simulink model "QRLsim"  (R2013b)
settings: Solver=ode3  StartTime=0.0  StopTime=Tsim_end  FixedStep=Tsim_s  RelTol=1e-3
values from neighbouring files (symbols this model uses):
  b = 0.1    [QRLrunfile.m]    (also in hat.m = vec(2))
  b1d = [1; 0; 0]    [QRLrunfile.m]
  ctauf = 8.004e-3    (= 0.008004)    [QRLrunfile.m]
  d = 0.1    [QRLrunfile.m]
  dq0 = [0;0;0]    [QRLrunfile.m]
  dxL0 = 0    [QRLrunfile.m]
  dyL0 = 0    [QRLrunfile.m]
  dzL0 = 0    [QRLrunfile.m]
  e3 = [0;0;1]    [QRLrunfile.m]
  fsat = inf*[1 -1]    [QRLrunfile.m]
  g = 9.81    [LQRrunfile.m]    (also in QRLrunfile.m)
  I = diag([Ixx Iyy Izz])    [QRLrunfile.m]
  Ir = 0.5    [QRLrunfile.m]
  Ixx = 0.0820    (= 0.082)    [LQRrunfile.m]    (also in QRLrunfile.m = 0.00223)
  Iyy = 0.0845    [LQRrunfile.m]    (also in QRLrunfile.m = 0.00299)
  Izz = 0.1377    [LQRrunfile.m]    (also in QRLrunfile.m = 0.0048)
  K = lqr(LQRA,LQRB,LQRQ,LQRR)    [LQRrunfile.m]
  kdx = facx*3    (= 3)    [QRLrunfile.m]
  komega = 0.1    [QRLQRATT-18-Apr-2017.mat]    (also in QRLrunfile.m = 0.75; savename.mat)
  kOmega = 0.4*facR    (= 0.04)    [QRLrunfile.m]
  kpx = facx*28.5    (= 28.5)    [QRLrunfile.m]
  kq = 4    [QRLQRATT-18-Apr-2017.mat]    (also in QRLrunfile.m = 2.25; savename.mat)
  kR = 8.81    [QRLQRATT-18-Apr-2017.mat]    (also in QRLrunfile.m = 0.285; savename.mat)
  L = 0.7    [QRLrunfile.m]
  l = 0.126    [QRLrunfile.m]
  LQRA = [zeros(8) eye(8) ... (first row only)    [LQRrunfile.m]
  LQRB = [zeros(10,4) ... (first row only)    [LQRrunfile.m]
  LQRC = eye(16)    [LQRrunfile.m]
  mL = 0.1    [LQRrunfile.m]    (also in QRLrunfile.m)
  mode = 4    [QRLrunfile.m]
  mQ = 4.34    [LQRrunfile.m]    (also in QRLrunfile.m = 0.4)
  Msat = inf*[1 -1]    [QRLrunfile.m]
  phiL0 = deg2rad(0)    [QRLrunfile.m]
  pQ0 = 0    [QRLrunfile.m]
  psiL0 = 0    [QRLrunfile.m]
  q0 = [0 0 -1]    [QRLQRATT-18-Apr-2017.mat]    (also in QRLrunfile.m = Rzyx*e3*qmode; savename.mat)
  qd = [0; 0; qmode]    [QRLrunfile.m]
  qmode = -1    [QRLrunfile.m]
  qQ0 = 0    [QRLrunfile.m]
  R0 = [1  0  0; 0  0.5  -0.866025403784; 0  0.866025403784  0.5]    [QRLQRATT-18-Apr-2017.mat]    (also in QRLrunfile.m = Rzyx; savename.mat)
  Rd = eye(3)    [QRLrunfile.m]
  rQ0 = 0    [QRLrunfile.m]
  stepamp = 0.25    [QRLrunfile.m]
  stept = 1.5    [QRLrunfile.m]
  T0 = 3    [QRLrunfile.m]
  thetaL0 = deg2rad(0)    [QRLrunfile.m]
  xL0 = q0(1)*L    [QRLrunfile.m]
  yL0 = q0(2)*L    [QRLrunfile.m]
  zL0 = L+q0(3)*L    [QRLrunfile.m]
undefined symbols (not defined in the file or in its folder): lqr0, sigbuilder_block
libraries: simulink_extras x8, CF3 x7, vrlib x5, simulink x5, dspmathops x4, aerolibtransform2 x2, CommandFilter x1
(part 1 of 2)
settings Model: Creator=Nam  LastModifiedBy=Nam
settings DataIOCC: SaveFormat=StructureWithTime
settings DebuggingCC: SolverPrmCheckMsg=none

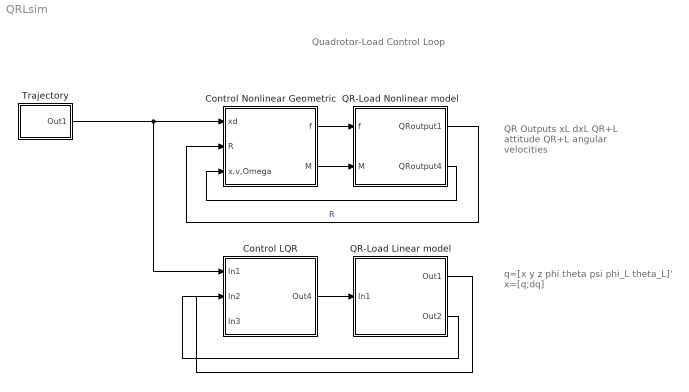
== system QRLsim ==
  note: Quadrotor-Load Control Loop
  note: QR Outputs
      | xL dxL
      | QR+L attitude
      | QR+L angular velocities
  note: q=[x y z phi theta psi phi_L theta_L]'
      | x=[q;dq]
  Control LQR : Subsystem
  Control Nonlinear Geometric : Subsystem
  QR-Load Linear model : Subsystem
  QR-Load Nonlinear model : Subsystem
  Trajectory : Subsystem
  wires:
  QR-Load Nonlinear model/1(QRoutput1) -> Control Nonlinear Geometric/2(R)  "R"
  QR-Load Nonlinear model/2(QRoutput4) -> Control Nonlinear Geometric/3(x,v,Omega)
  Control Nonlinear Geometric/1(f) -> QR-Load Nonlinear model/1(f)
  Control Nonlinear Geometric/2(M) -> QR-Load Nonlinear model/2(M)
  QR-Load Linear model/2(Out2) -> Control LQR/2(In2)
  Control LQR/1(Out4) -> QR-Load Linear model/1(In1)
  Trajectory/1(Out1) -> Control Nonlinear Geometric/1(xd), Control LQR/1(In1)
  QR-Load Linear model/1(Out1) -> ?

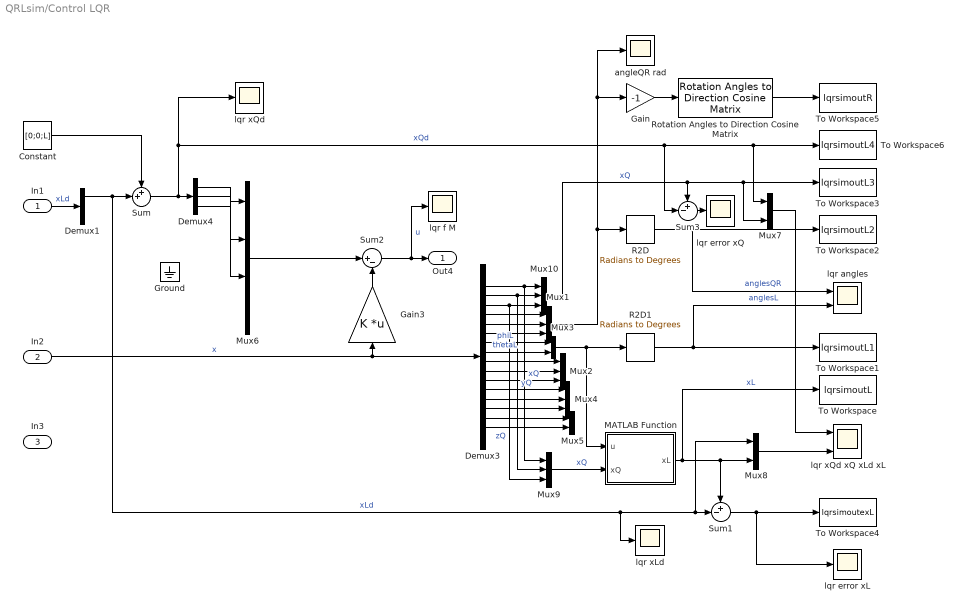
== system QRLsim/Control LQR ==
  In1 : Inport
  In2 : Inport  Port=2
  In3 : Inport  Port=3
  Constant : Constant  Value=[0;0;L]
  Demux1 : Demux  Outputs=3
  Demux3 : Demux  Outputs=16
  Demux4 : Demux  Outputs=3
  Gain : Gain  Gain=-1
  Gain3 : Gain  Gain=K  Multiplication=Matrix(K*u)
  Ground : Ground
  MATLAB Function : MATLAB Function  TreatAsAtomicUnit=on
  Mux{1..2,4,9..10} (5 alike) : Mux  Inputs=3
  Mux{3,5,7..8} (4 alike) : Mux  Inputs=2
  Mux6 : Mux
  R2D : simulink_extras/Transformations/Radians to Degrees
  R2D1 : simulink_extras/Transformations/Radians to Degrees
  Rotation Angles to Direction Cosine Matrix : aerolibtransform2/Rotation Angles to Direction Cosine Matrix  rotationOrder=XYZ
  Sum : Sum  Inputs=++|
  Sum1 : Sum  Inputs=+-|
  Sum2 : Sum  Inputs=|+-
  Sum3 : Sum  Inputs=+-|
  To Workspace : ToWorkspace  VariableName=lqrsimoutL  SampleTime=-1  SaveFormat=Structure With Time
  To Workspace1 : ToWorkspace  VariableName=lqrsimoutL1  SampleTime=-1  SaveFormat=Structure With Time
  To Workspace2 : ToWorkspace  VariableName=lqrsimoutL2  SampleTime=-1  SaveFormat=Structure With Time
  To Workspace3 : ToWorkspace  VariableName=lqrsimoutL3  SampleTime=-1  SaveFormat=Structure With Time
  To Workspace4 : ToWorkspace  VariableName=lqrsimoutexL  SampleTime=-1  SaveFormat=Structure With Time
  To Workspace5 : ToWorkspace  VariableName=lqrsimoutR  SampleTime=-1  SaveFormat=Structure With Time
  To Workspace6 : ToWorkspace  VariableName=lqrsimoutL4  SampleTime=-1  SaveFormat=Structure With Time
  angleQR rad : Scope
      settings: TimeRange=25  YMin=-0.3  YMax=1.1  SaveName=ScopeData20
  lqr angles : Scope  NumInputPorts=2
      settings: TimeRange=20  YMin=-30~-40  YMax=30~40  SaveName=ScopeData11
  lqr error xL : Scope
      settings: TimeRange=20  YMin=-1.5  YMax=2
  lqr error xQ : Scope
      settings: TimeRange=25  YMin=-0.25  YMax=0.1  SaveName=ScopeData18
  lqr f M : Scope
      settings: ShowLegends=on  SaveName=ScopeData13
  lqr xLd : Scope
      settings: TimeRange=25  YMin=-0.3  YMax=1.1  SaveName=ScopeData56
  lqr xQd : Scope
      settings: TimeRange=25  YMin=-0.25  YMax=0.1  SaveName=ScopeData58
  lqr xQd xQ xLd xL : Scope  NumInputPorts=2
      settings: ShowLegends=on  TimeRange=20  YMin=-1.5~-2  YMax=1.5~2  SaveName=ScopeData14
  Out4 : Outport
  wires:
  Constant/1 -> Sum/1
  Mux10/1 -> Mux7/2, To Workspace3/1, Sum3/1  "xQ"
  Demux1/1 -> Sum/2, lqr xLd/1, Sum1/2, Mux8/1  "xLd"
  Demux3/12 -> Mux4/1
  Demux3/14 -> Mux4/3
  Demux3/8 -> Mux3/2  "thetaL"
  Demux3/5 -> Mux1/2
  Demux3/13 -> Mux4/2
  Demux3/2 -> Mux10/2, Mux9/2  "yQ"
  Mux3/1 -> MATLAB Function/1(u), R2D1/1
  R2D/1 -> lqr angles/1, To Workspace2/1  "anglesQR"
  Sum/1 -> lqr xQd/1, Mux7/1, To Workspace6/1, Sum3/2, Demux4/1  "xQd"
  Demux3/3 -> Mux10/3, Mux9/3  "zQ"
  Mux1/1 -> angleQR rad/1, Gain/1, R2D/1
  Mux9/1 -> MATLAB Function/2(xQ)  "xQ"
  Mux6/1 -> Sum2/1
  Demux3/1 -> Mux10/1, Mux9/1  "xQ"
  MATLAB Function/1(xL) -> Sum1/1, Mux8/2, To Workspace/1  "xL"
  Demux3/15 -> Mux5/1
  Demux3/4 -> Mux1/1
  Demux3/16 -> Mux5/2
  Demux3/7 -> Mux3/1  "phiL"
  Demux3/6 -> Mux1/3
  Demux3/11 -> Mux2/3
  Demux3/10 -> Mux2/2
  Demux3/9 -> Mux2/1
  In1/1 -> Demux1/1  "xLd"
  Sum2/1 -> Out4/1, lqr f M/1  "u"
  In2/1 -> Demux3/1, Gain3/1  "x"
  Sum1/1 -> lqr error xL/1, To Workspace4/1
  R2D1/1 -> To Workspace1/1, lqr angles/2  "anglesL"
  Mux8/1 -> lqr xQd xQ xLd xL/2
  Mux7/1 -> lqr xQd xQ xLd xL/1
  Sum3/1 -> lqr error xQ/1
  Rotation Angles to Direction Cosine Matrix/1 -> To Workspace5/1
  Gain/1 -> Rotation Angles to Direction Cosine Matrix/1
  Demux4/1 -> Mux6/1
  Demux4/2 -> Mux6/2
  Demux4/3 -> Mux6/3
  Gain3/1 -> Sum2/2

== system QRLsim/Control Nonlinear Geometric ==
  note: Control
  xd : Inport
  R : Inport  Port=2
  x,v,Omega : Inport  Port=3
  QRL Load Attitude Controller : Subsystem
  QRL Load Position Controller : Subsystem
  QRL QR Attitude Controller : Subsystem
  f : Outport
  M : Outport  Port=2
  wires:
  R/1 -> QRL Load Attitude Controller/3(R), QRL QR Attitude Controller/4(R1)
  x,v,Omega/1 -> QRL Load Attitude Controller/4(QROutput), QRL QR Attitude Controller/5(Omega), QRL Load Position Controller/2(QROutput1)
  xd/1 -> QRL Load Position Controller/1(xdes)
  QRL QR Attitude Controller/1(M) -> M/1  "M"
  QRL Load Attitude Controller/2(b3d2) -> QRL QR Attitude Controller/1(R)
  QRL Load Position Controller/1(b3d1) -> QRL Load Attitude Controller/1(xdes1)
  QRL Load Position Controller/2(f) -> QRL Load Attitude Controller/2(R1)
  QRL Load Attitude Controller/1(b3d1) -> f/1  "f"
  QRL Load Attitude Controller/3(b3d3) -> QRL QR Attitude Controller/2(R2)
  QRL Load Attitude Controller/4(b3d4) -> QRL QR Attitude Controller/3(R3)

== system QRLsim/QR-Load Linear model ==
  In1 : Inport
  Gain1 : Gain  Gain=LQRA  Multiplication=Matrix(K*u)
  Gain2 : Gain  Gain=LQRB  Multiplication=Matrix(K*u)
  Gain5 : Gain  Gain=LQRC  Multiplication=Matrix(K*u)
  Integrator : Integrator  InitialCondition=lqr0
  Sum1 : Sum  Inputs=|++
  Out1 : Outport
  Out2 : Outport  Port=2
  wires:
  Gain1/1 -> Sum1/2
  Sum1/1 -> Integrator/1  "dx"
  Integrator/1 -> Gain1/1, Out2/1, Gain5/1  "x"
  Gain2/1 -> Sum1/1
  In1/1 -> Gain2/1  "u"
  Gain5/1 -> Out1/1  "y"

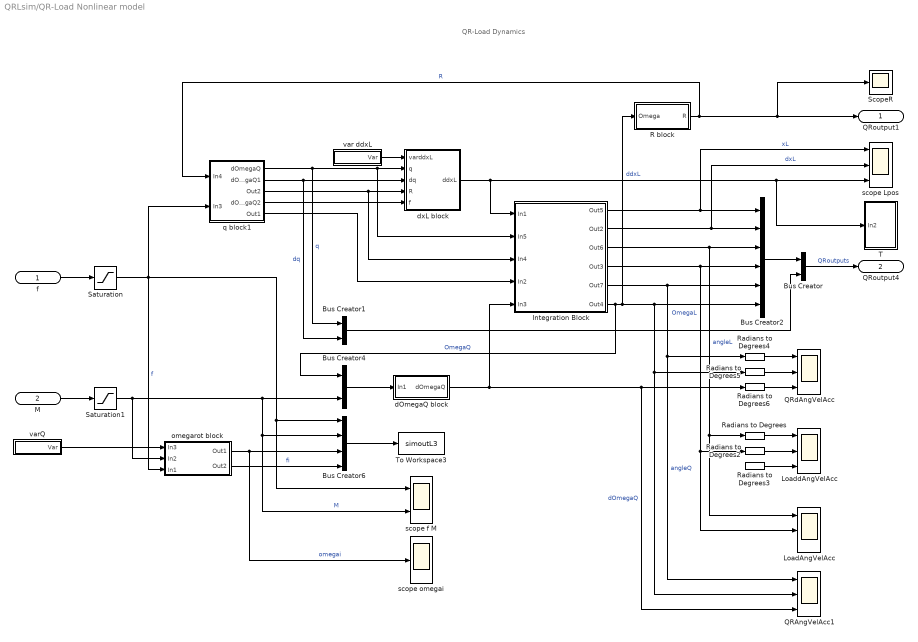
== system QRLsim/QR-Load Nonlinear model ==
  note: QR-Load Dynamics
  f : Inport
  M : Inport  Port=2  PortDimensions=3
  Bus Creator : BusCreator  Inputs=2
  Bus Creator1 : BusCreator  Inputs=2
  Bus Creator2 : BusCreator  Inputs=6
  Bus Creator4 : BusCreator  Inputs=2
  Bus Creator6 : BusCreator
  Integration Block : Subsystem
  LoadAngVelAcc : Scope  NumInputPorts=3
      settings: ShowLegends=on  YMin=-0.65~-20~-2000  YMax=0.15~12.5~1000  SaveName=ScopeData10
  LoaddAngVelAcc : Scope  NumInputPorts=3
      settings: ShowLegends=on  YMin=-5~-5~-5  YMax=5~5~5  SaveName=ScopeData4
  QRAngVelAcc1 : Scope  NumInputPorts=3
      settings: ShowLegends=on  YMin=-0.65~-20~-2000  YMax=0.15~12.5~1000  SaveName=ScopeData15
  QRdAngVelAcc : Scope  NumInputPorts=3
      settings: ShowLegends=on  TimeRange=20  YMin=-60~-600~-15000  YMax=60~800~20000  SaveName=ScopeData3
  R block : Subsystem
  Radians to Degrees{,2..6} (6 alike) : simulink_extras/Transformations/Radians to Degrees
  Saturation : Saturate  UpperLimit=fsat(1)  LowerLimit=fsat(2)
  Saturation1 : Saturate  UpperLimit=Msat(1)  LowerLimit=Msat(2)
  ScopeR : Scope
      settings: SaveName=ScopeData37
  T : Subsystem
  To Workspace3 : ToWorkspace  VariableName=simoutL3  SampleTime=-1  SaveFormat=Structure With Time
  dOmegaQ block : Subsystem
  dxL block : MATLAB Function  TreatAsAtomicUnit=on
  omegarot block : Subsystem
      mask Display: disp('(f,M) \rightarrow (\omega_i,f_i)','texmode','on')
  q block1 : Subsystem
  scope Lpos : Scope  NumInputPorts=3
      settings: ShowLegends=on  TimeRange=30  YMin=0~0~-100  YMax=7~6~250  SaveName=ScopeData12
  scope f M : Scope  NumInputPorts=2
      settings: ShowLegends=on  TimeRange=10  YMin=4.65~-2.25  YMax=5.35~1.25  SaveName=ScopeData42
  scope omegai : Scope
      settings: ShowLegends=on  YMin=42  YMax=54  SaveName=ScopeData16
  var ddxL : Subsystem
  varQ : Subsystem
  QRoutput1 : Outport
  QRoutput4 : Outport  Port=2
  wires:
  dxL block/1(ddxL) -> Integration Block/1(In1), T/1(In2), scope Lpos/3  "ddxL"
  dOmegaQ block/1(dOmegaQ) -> Integration Block/5(In3), Radians to Degrees6/1, QRAngVelAcc1/3  "dOmegaQ"
  Bus Creator4/1 -> dOmegaQ block/1(In1)
  M/1 -> Saturation1/1
  var ddxL/1(Var) -> dxL block/1(varddxL)
  q block1/2(dOmegaQ1) -> Bus Creator1/2, dxL block/3(dq)  "dq"
  q block1/3(Out2) -> dxL block/4(R), Integration Block/3(In4)
  q block1/1(dOmegaQ) -> Bus Creator1/1, Integration Block/2(In5), dxL block/2(q)  "q"
  Integration Block/5(Out7) -> Bus Creator2/5, Radians to Degrees4/1, QRAngVelAcc1/1  "angleQ"
  Integration Block/2(Out2) -> Bus Creator2/2, scope Lpos/2  "dxL"
  Integration Block/4(Out3) -> Bus Creator2/4, LoadAngVelAcc/2, Radians to Degrees2/1  "OmegaL"
  Integration Block/6(Out4) -> Bus Creator2/6, Radians to Degrees5/1, QRAngVelAcc1/2, R block/1(Omega), Bus Creator4/1  "OmegaQ"
  Integration Block/1(Out5) -> Bus Creator2/1, scope Lpos/1  "xL"
  varQ/1(Var) -> omegarot block/1(In3)
  Integration Block/3(Out6) -> Bus Creator2/3, LoadAngVelAcc/1, Radians to Degrees/1  "angleL"
  Bus Creator6/1 -> To Workspace3/1
  Radians to Degrees/1 -> LoaddAngVelAcc/1
  Radians to Degrees2/1 -> LoaddAngVelAcc/2
  Radians to Degrees3/1 -> LoaddAngVelAcc/3
  Radians to Degrees5/1 -> QRdAngVelAcc/2
  Radians to Degrees4/1 -> QRdAngVelAcc/1
  Radians to Degrees6/1 -> QRdAngVelAcc/3
  R block/1(R) -> QRoutput1/1, ScopeR/1, q block1/1(In4)  "R"
  Bus Creator1/1 -> Bus Creator/2
  Bus Creator2/1 -> Bus Creator/1
  Bus Creator/1 -> QRoutput4/1  "QRoutputs"
  q block1/5(Out1) -> Integration Block/4(In2)
  f/1 -> Saturation/1
  omegarot block/1(Out1) -> scope omegai/1, Bus Creator6/3  "omegai"
  Saturation/1 -> scope f M/1, Bus Creator6/1, q block1/2(In3), omegarot block/3(In1)  "f"
  Saturation1/1 -> omegarot block/2(In2), Bus Creator4/2, scope f M/2, Bus Creator6/2  "M"
  omegarot block/2(Out2) -> Bus Creator6/4  "fi"
  q block1/4(dOmegaQ2) -> dxL block/5(f)

== system QRLsim/Trajectory ==
  Command Filter1 : CF3/Command Filter  Integrator1_init=0  omega_n1=omega_n1_xL  omega_n2=omega_n2_xL  zeta=zeta_xL
  Ellipse : Subsystem
  Manual Switch : ManualSwitch
  Manual Switch1 : ManualSwitch
  Mux2 : Mux  Inputs=3
  Path : Subsystem
  Scope2 : Scope  NumInputPorts=3
      settings: ShowLegends=on  TimeRange=25  YMin=-0.5~-0.8~-5  YMax=2~0.6000000000000001~5
  Step : Subsystem
  Terminator : Terminator
  Out1 : Outport
  wires:
  Command Filter1/3 -> Scope2/2, Mux2/2
  Command Filter1/4 -> Scope2/3, Mux2/3
  Command Filter1/2 -> Terminator/1
  Command Filter1/1 -> Scope2/1, Mux2/1
  Mux2/1 -> Out1/1
  Manual Switch1/1 -> Command Filter1/1  "xLd"
  Step/1(Out2) -> Manual Switch/1
  Path/1(Out3) -> Manual Switch/2
  Manual Switch/1 -> Manual Switch1/1
  Ellipse/1(Out3) -> Manual Switch1/2

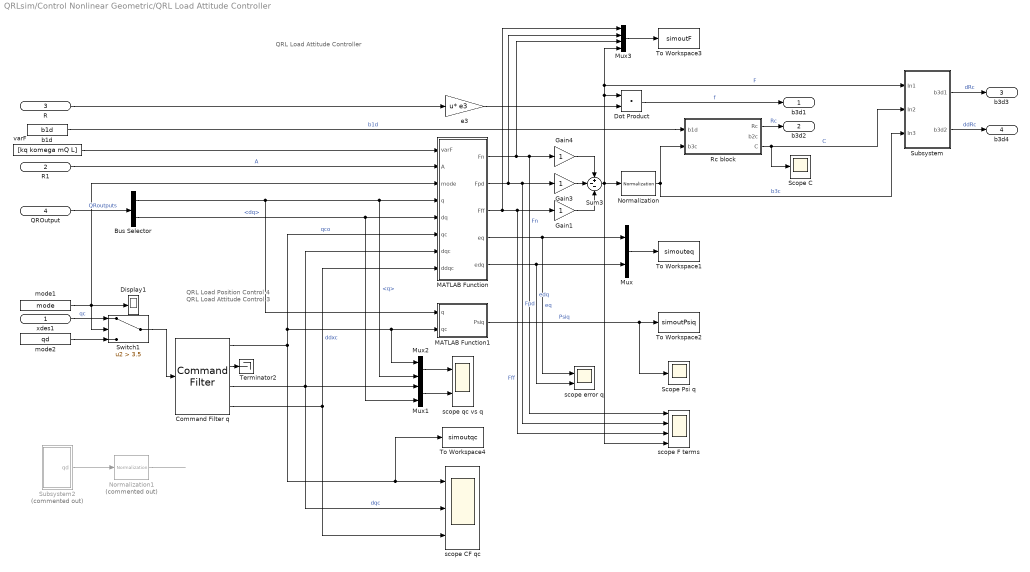
== system QRLsim/Control Nonlinear Geometric/QRL Load Attitude Controller ==
  note: QRL Load Attitude Controller
  note: QRL Load Position Control 4
      | QRL Load Attitude Control 3
  xdes1 : Inport
  R1 : Inport  Port=2
  R : Inport  Port=3
  QROutput : Inport  Port=4
  Bus Selector : BusSelector  OutputSignals=signal2.q,signal2.dq
  Command Filter q : CF3/Command Filter  Integrator1_init=q0  omega_n1=omega_n1_q  omega_n2=omega_n2_q  zeta=zeta_q
  Display1 : Display
  Dot Product : DotProduct  InputSameDT=on  OutDataTypeStr=Inherit: Inherit via internal rule
  Gain1 : Gain
  Gain3 : Gain
  Gain4 : Gain
  MATLAB Function : MATLAB Function  TreatAsAtomicUnit=on
  MATLAB Function1 : MATLAB Function  TreatAsAtomicUnit=on
  Mux : Mux  Inputs=2
  Mux1 : Mux  Inputs=2
  Mux2 : Mux  Inputs=2
  Mux3 : Mux
  Normalization : dspmathops/Normalization  NormType=2-norm  Bias=1e-10  NormOver=Each column  ColComp=on  Dimension=1  outputDataTypeStr=Inherit: Same as product output  outputLastDataTypeStr=Inherit: Same as product output  outputMin=[]  outputMax=[]  accumDataTypeStr=Inherit: Same as product output  accumLastDataTypeStr=Inherit: Same as product output  roundingMode=Floor  overflowMode=off
  Normalization1 : dspmathops/Normalization  Commented=on  NormType=2-norm  Bias=1e-10  NormOver=Each column  ColComp=on  Dimension=1  outputDataTypeStr=Inherit: Same as product output  outputLastDataTypeStr=Inherit: Same as product output  outputMin=[]  outputMax=[]  accumDataTypeStr=Inherit: Same as product output  accumLastDataTypeStr=Inherit: Same as product output  roundingMode=Floor  overflowMode=off
  Rc block : MATLAB Function  TreatAsAtomicUnit=on
  Scope C : Scope
      settings: ShowLegends=on  TimeRange=30  YMin=0  YMax=0.003  SaveName=ScopeData26
  Scope Psi q : Scope
      settings: ShowLegends=on  TimeRange=30  YMin=0  YMax=0.003  SaveName=ScopeData47
  Subsystem : Subsystem
  Subsystem2 : Subsystem  Commented=on
  Sum3 : Sum  Inputs=+--
  Switch1 : Switch  Criteria=u2 > Threshold  Threshold=3.5
  Terminator2 : Terminator
  To Workspace1 : ToWorkspace  VariableName=simouteq  SampleTime=-1  SaveFormat=Structure With Time
  To Workspace2 : ToWorkspace  VariableName=simoutPsiq  SampleTime=-1  SaveFormat=Structure With Time
  To Workspace3 : ToWorkspace  VariableName=simoutF  SampleTime=-1  SaveFormat=Structure With Time
  To Workspace4 : ToWorkspace  VariableName=simoutqc  SampleTime=-1  SaveFormat=Structure With Time
  b1d : Constant  Value=b1d  VectorParams1D=off
  e3 : Gain  Gain=e3  Multiplication=Matrix(u*K)
  mode1 : Constant  Value=mode  VectorParams1D=off
  mode2 : Constant  Value=qd  VectorParams1D=off
  scope CF qc : Scope  NumInputPorts=3
      settings: ShowLegends=on  YMin=-1~-1.5~-40  YMax=0.5~0.5~60  SaveName=ScopeData19
  scope F terms : Scope  NumInputPorts=4
      settings: TimeRange=15  YMin=-5~-5~-5~-5  YMax=5~5~5~5  SaveName=ScopeData31
  scope error q : Scope  NumInputPorts=2
      settings: TimeRange=10  YMin=-0.14~-0.5  YMax=0.06~0.5  SaveName=ScopeData33
  scope qc vs q : Scope  NumInputPorts=2
      settings: ShowLegends=on  TimeRange=10  YMin=-1~-1  YMax=0.4000000000000001~0.8  SaveName=ScopeData46
  varF : Constant  Value=[kq komega mQ L]  VectorParams1D=off
  b3d1 : Outport
  b3d2 : Outport  Port=2
  b3d3 : Outport  Port=3
  b3d4 : Outport  Port=4
  wires:
  Rc block/1(Rc) -> b3d2/1  "Rc"
  Normalization/1 -> Subsystem/3(In3), Rc block/2(b3c)  "b3c"
  b1d/1 -> Rc block/1(b1d)  "b1d"
  Sum3/1 -> Dot Product/1, Mux3/4, Subsystem/1(In1), Normalization/1, scope F terms/4  "F"
  mode1/1 -> Switch1/2, MATLAB Function/3(mode), Display1/1
  Command Filter q/1 -> MATLAB Function/6(qc), Mux2/1, MATLAB Function1/2(qc), scope CF qc/1, To Workspace4/1  "qco"
  QROutput/1 -> Bus Selector/1  "QRoutputs"
  MATLAB Function/3(Fff) -> Mux3/1, Gain1/1, scope F terms/3  "Fff"
  MATLAB Function/2(Fpd) -> Mux3/2, Gain3/1, scope F terms/2  "Fpd"
  MATLAB Function/1(Fn) -> Mux3/3, Gain4/1, scope F terms/1  "Fn"
  Bus Selector/1 -> Mux2/2, MATLAB Function/4(q), MATLAB Function1/1(q)  "<q>"
  Bus Selector/2 -> MATLAB Function/5(dq), Mux1/2  "<dq>"
  varF/1 -> MATLAB Function/1(varF)
  MATLAB Function1/1(Psiq) -> Scope Psi q/1, To Workspace2/1  "Psiq"
  Dot Product/1 -> b3d1/1  "f"
  e3/1 -> Dot Product/2
  R/1 -> e3/1
  MATLAB Function/5(edq) -> Mux/2, scope error q/2  "edq"
  MATLAB Function/4(eq) -> Mux/1, scope error q/1  "eq"
  Mux/1 -> To Workspace1/1
  R1/1 -> MATLAB Function/2(A)  "A"
  Gain1/1 -> Sum3/3
  mode2/1 -> Switch1/3
  Normalization1/1 -> ?
  Gain3/1 -> Sum3/2
  Gain4/1 -> Sum3/1
  Command Filter q/3 -> scope CF qc/2, Mux1/1, MATLAB Function/7(dqc)  "dqc"
  Command Filter q/4 -> scope CF qc/3, MATLAB Function/8(ddqc)  "ddxc"
  Mux2/1 -> scope qc vs q/1
  Mux1/1 -> scope qc vs q/2
  Subsystem2/1(qd) -> Normalization1/1
  Switch1/1 -> Command Filter q/1
  Command Filter q/2 -> Terminator2/1
  Mux3/1 -> To Workspace3/1
  xdes1/1 -> Switch1/1  "qc"
  Rc block/3(C) -> Scope C/1, Subsystem/2(In2)  "C"
  Subsystem/1(b3d1) -> b3d3/1  "dRc"
  Subsystem/2(b3d2) -> b3d4/1  "ddRc"

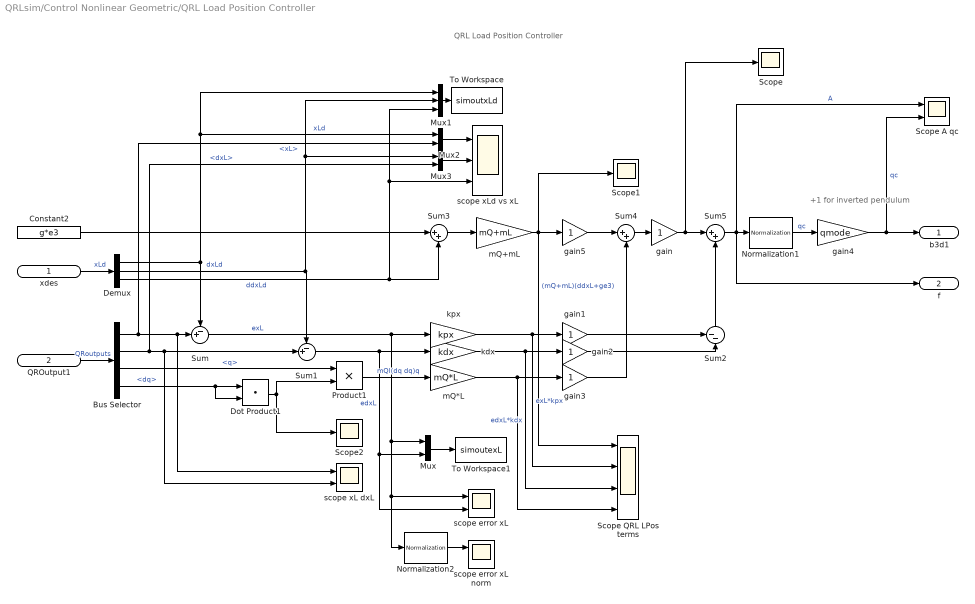
== system QRLsim/Control Nonlinear Geometric/QRL Load Position Controller ==
  note: +1 for
      | inverted pendulum
  note: QRL Load Position Controller
  xdes : Inport
  QROutput1 : Inport  Port=2
  Bus Selector : BusSelector  OutputSignals=signal1.xL,signal1.dxL,signal2.q,signal2.dq
  Constant2 : Constant  Value=g*e3
  Demux : Demux  Outputs=3
  Dot Product1 : DotProduct  InputSameDT=on  OutDataTypeStr=Inherit: Inherit via internal rule
  Mux : Mux  Inputs=2
  Mux1 : Mux  Inputs=3
  Mux2 : Mux  Inputs=2
  Mux3 : Mux  Inputs=2
  Normalization1 : dspmathops/Normalization  NormType=2-norm  Bias=1e-10  NormOver=Each column  ColComp=on  Dimension=1  outputDataTypeStr=Inherit: Same as product output  outputLastDataTypeStr=Inherit: Same as product output  outputMin=[]  outputMax=[]  accumDataTypeStr=Inherit: Same as product output  accumLastDataTypeStr=Inherit: Same as product output  roundingMode=Floor  overflowMode=off
  Normalization2 : dspmathops/Normalization  NormType=2-norm  Bias=1e-10  NormOver=Each column  ColComp=on  Dimension=1  outputDataTypeStr=Inherit: Same as product output  outputLastDataTypeStr=Inherit: Same as product output  outputMin=[]  outputMax=[]  accumDataTypeStr=Inherit: Same as product output  accumLastDataTypeStr=Inherit: Same as product output  roundingMode=Floor  overflowMode=off
  Product1 : Product
  Scope : Scope
      settings: ShowLegends=on  SaveName=ScopeData35
  Scope A qc : Scope  NumInputPorts=2
      settings: ShowLegends=on  YMin=-5~-5  YMax=5~5  SaveName=ScopeData34
  Scope QRL LPos terms : Scope  NumInputPorts=4
      settings: YMin=-5~-5~-5~-5  YMax=5~5~5~5  SaveName=ScopeData32
  Scope1 : Scope
      settings: ShowLegends=on  SaveName=ScopeData36
  Scope2 : Scope
      settings: ShowLegends=on  SaveName=ScopeData25
  Sum : Sum  Inputs=-+|
  Sum1 : Sum  Inputs=-+|
  Sum2 : Sum  Inputs=--|
  Sum3 : Sum  Inputs=|++
  Sum4 : Sum  Inputs=|++
  Sum5 : Sum  Inputs=|++
  To Workspace : ToWorkspace  VariableName=simoutxLd  SampleTime=-1  SaveFormat=Structure With Time
  To Workspace1 : ToWorkspace  VariableName=simoutexL  SampleTime=-1  SaveFormat=Structure With Time
  gain{,1..3,5} (5 alike) : Gain
  gain4 : Gain  Gain=qmode
  kdx : Gain  Gain=kdx
  kpx : Gain  Gain=kpx
  mQ*L : Gain  Gain=mQ*L
  mQ+mL : Gain  Gain=mQ+mL
  scope error xL : Scope  NumInputPorts=2
      settings: ShowLegends=on  TimeRange=10  YMin=-0.01~-0.06  YMax=0.05~0.12  SaveName=ScopeData28
  scope error xL norm : Scope  NumInputPorts=2
      settings: ShowLegends=on  TimeRange=15  YMin=-1~-200  YMax=1~275  SaveName=ScopeData57
  scope xL dxL : Scope  NumInputPorts=2
      settings: TimeRange=20  YMin=-0.5~-0.4  YMax=3.5~1.6  SaveName=ScopeData40
  scope xLd vs xL : Scope  NumInputPorts=3
      settings: ShowLegends=on  TimeRange=10  YMin=-0.025~-0.2~-0.75  YMax=0.3~0.4~0.75  SaveName=ScopeData41
  b3d1 : Outport
  f : Outport  Port=2
  wires:
  QROutput1/1 -> Bus Selector/1  "QRoutputs"
  Sum/1 -> kpx/1, Mux/1, Normalization2/1, scope error xL/1  "exL"
  Sum1/1 -> Mux/2, scope error xL/2, kdx/1  "edxL"
  Bus Selector/1 -> Mux2/2, scope xL dxL/1, Sum/2  "<xL>"
  Bus Selector/2 -> Mux3/2, scope xL dxL/2, Sum1/2  "<dxL>"
  Sum5/1 -> Scope A qc/1, f/1, Normalization1/1  "A"
  Constant2/1 -> Sum3/1
  Sum3/1 -> mQ+mL/1
  mQ+mL/1 -> gain5/1, Scope1/1, Scope QRL LPos terms/1  "(mQ+mL)(ddxL+ge3)"
  kpx/1 -> gain1/1, Scope QRL LPos terms/2  "exL*kpx"
  kdx/1 -> Scope QRL LPos terms/3, gain2/1  "edxL*kdx"
  Bus Selector/3 -> Product1/1  "<q>"
  Bus Selector/4 -> Dot Product1/2, Dot Product1/1  "<dq>"
  Dot Product1/1 -> Product1/2, Scope2/1
  Product1/1 -> mQ*L/1  "mQl(dq dq)q"
  Mux/1 -> To Workspace1/1
  Normalization1/1 -> gain4/1  "qc"
  gain3/1 -> Sum4/2
  gain4/1 -> Scope A qc/2, b3d1/1  "qc"
  gain2/1 -> Sum2/2
  gain1/1 -> Sum2/1
  Sum2/1 -> Sum5/2
  Sum4/1 -> gain/1
  gain/1 -> Scope/1, Sum5/1
  Mux1/1 -> To Workspace/1
  xdes/1 -> Demux/1  "xLd"
  Demux/1 -> Sum/1, Mux1/1, Mux2/1  "xLd"
  Demux/2 -> Mux1/2, Mux3/1, Sum1/1  "dxLd"
  Demux/3 -> Sum3/2, Mux1/3, scope xLd vs xL/3  "ddxLd"
  Mux2/1 -> scope xLd vs xL/1
  Mux3/1 -> scope xLd vs xL/2
  gain5/1 -> Sum4/1
  Normalization2/1 -> scope error xL norm/1
  mQ*L/1 -> Scope QRL LPos terms/4, gain3/1

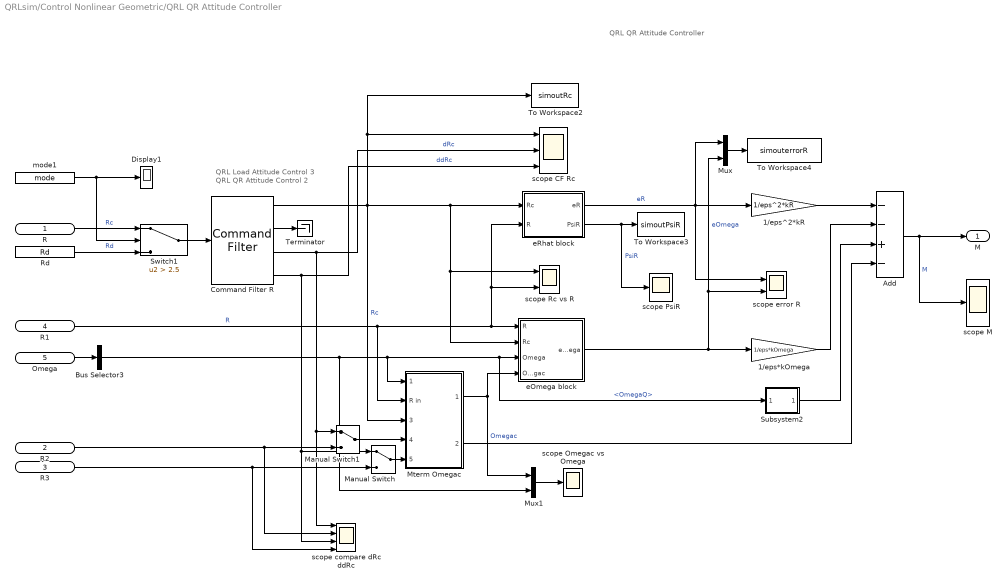
== system QRLsim/Control Nonlinear Geometric/QRL QR Attitude Controller ==
  note: QRL QR Attitude Controller
  note: QRL Load Attitude Control 3
      | QRL QR Attitude Control 2
  R : Inport
  R2 : Inport  Port=2
  R3 : Inport  Port=3
  R1 : Inport  Port=4
  Omega : Inport  Port=5
  1/eps*kOmega : Gain  Gain=1/eps*kOmega
  1/eps^2*kR : Gain  Gain=1/eps^2*kR
  Add : Sum  Inputs=--+-
  Bus Selector3 : BusSelector  OutputSignals=signal1.OmegaQ
  Command Filter R : CF3/Command Filter  Integrator1_init=R0  omega_n1=omega_n1_R  omega_n2=omega_n2_R  zeta=zeta_R
  Display1 : Display
  Manual Switch : ManualSwitch
  Manual Switch1 : ManualSwitch
  Mterm Omegac : Subsystem
  Mux : Mux  Inputs=2
  Mux1 : Mux  Inputs=2
  Rd : Constant  Value=Rd  VectorParams1D=off
  Subsystem2 : Subsystem
      mask Display: disp('\Omega \times I\Omega','texmode','on')
  Switch1 : Switch  Criteria=u2 > Threshold  Threshold=2.5
  Terminator : Terminator
  To Workspace2 : ToWorkspace  VariableName=simoutRc  SampleTime=-1  SaveFormat=Structure With Time
  To Workspace3 : ToWorkspace  VariableName=simoutPsiR  SampleTime=-1  SaveFormat=Structure With Time
  To Workspace4 : ToWorkspace  VariableName=simouterrorR  SampleTime=-1  SaveFormat=Structure With Time
  eOmega block : MATLAB Function  TreatAsAtomicUnit=on
  eRhat block : MATLAB Function  TreatAsAtomicUnit=on
  mode1 : Constant  Value=mode  VectorParams1D=off
  scope CF Rc : Scope  NumInputPorts=3
      settings: ShowLegends=on  YMin=-5~-5~-5  YMax=5~5~5  SaveName=ScopeData49
  scope M : Scope
      settings: ShowLegends=on  SaveName=ScopeData5
  scope Omegac vs Omega : Scope
      settings: ShowLegends=on  TimeRange=20  YMin=-1  YMax=1  SaveName=ScopeData51
  scope PsiR : Scope
      settings: ShowLegends=on  TimeRange=30  YMin=0  YMax=0.0025  SaveName=ScopeData44
  scope Rc vs R : Scope  NumInputPorts=2
      settings: ShowLegends=on  TimeRange=10  YMin=-0.8~-0.8  YMax=1~1  SaveName=ScopeData48
  scope compare dRc ddRc : Scope  NumInputPorts=4
      settings: ShowLegends=on  TimeRange=20  YMin=-1~-5~-5~-5  YMax=1~5~5~5  SaveName=ScopeData6
  scope error R : Scope  NumInputPorts=2
      settings: ShowLegends=on  TimeRange=10  YMin=-0.8~-4  YMax=0.6000000000000001~4  SaveName=ScopeData30
  M : Outport  PortDimensions=3
  wires:
  mode1/1 -> Switch1/2, Display1/1
  R/1 -> Switch1/1  "Rc"
  Rd/1 -> Switch1/3  "Rd"
  R1/1 -> scope Rc vs R/2, eRhat block/2(R), eOmega block/1(R), Mterm Omegac/2(R in)  "R"
  Omega/1 -> Bus Selector3/1
  Bus Selector3/1 -> Mux1/2, Mterm Omegac/1(Omega in), Subsystem2/1(Omega), eOmega block/3(Omega)  "<OmegaQ>"
  eRhat block/1(eR) -> 1/eps^2*kR/1, scope error R/1, Mux/1  "eR"
  Mterm Omegac/1(Omegades) -> Mux1/1, eOmega block/4(Omegac)  "Omegac"
  eOmega block/1(eOmega) -> 1/eps*kOmega/1, scope error R/2, Mux/2  "eOmega"
  1/eps^2*kR/1 -> Add/1
  1/eps*kOmega/1 -> Add/2
  Subsystem2/1(Out1) -> Add/3
  Mterm Omegac/2(M term) -> Add/4
  Add/1 -> scope M/1, M/1  "M"
  eRhat block/2(PsiR) -> scope PsiR/1, To Workspace3/1  "PsiR"
  Mux/1 -> To Workspace4/1
  Command Filter R/3 -> Manual Switch1/1, scope compare dRc ddRc/1, scope CF Rc/2  "dRc"
  Command Filter R/4 -> Manual Switch/1, scope compare dRc ddRc/3, scope CF Rc/3  "ddRc"
  Command Filter R/1 -> Mterm Omegac/3(Rdes in), eRhat block/1(Rc), scope Rc vs R/1, eOmega block/2(Rc), To Workspace2/1, scope CF Rc/1  "Rc"
  Mux1/1 -> scope Omegac vs Omega/1
  Switch1/1 -> Command Filter R/1
  Command Filter R/2 -> Terminator/1
  R2/1 -> Manual Switch1/2, scope compare dRc ddRc/2
  R3/1 -> Manual Switch/2, scope compare dRc ddRc/4
  Manual Switch1/1 -> Mterm Omegac/4(Rdes in1)
  Manual Switch/1 -> Mterm Omegac/5(Rdes in2)

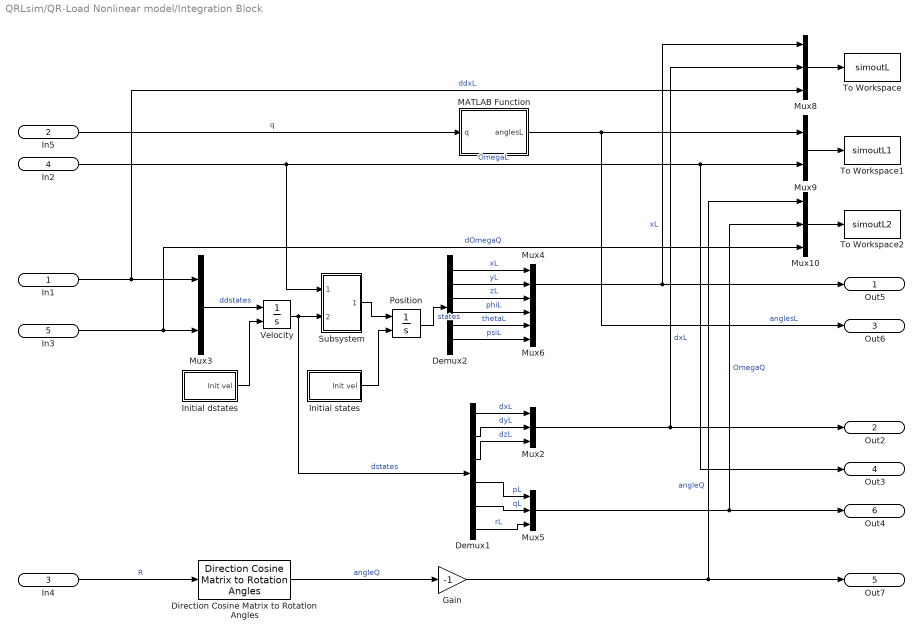
== system QRLsim/QR-Load Nonlinear model/Integration Block ==
  In1 : Inport
  In5 : Inport  Port=2
  In4 : Inport  Port=3
  In2 : Inport  Port=4
  In3 : Inport  Port=5
  Demux1 : Demux  Outputs=6
  Demux2 : Demux  Outputs=6
  Direction Cosine Matrix to Rotation Angles : aerolibtransform2/Direction Cosine Matrix to Rotation Angles  rotationOrder=XYZ  lim=Default
      settings: AttributesFormatString=Rotation Order: %<rotationOrder>
  Gain : Gain  Gain=-1
  Initial dstates : Subsystem
  Initial states : Subsystem
  MATLAB Function : MATLAB Function  TreatAsAtomicUnit=on
  Mux{2,4..6,8,10} (6 alike) : Mux  Inputs=3
  Mux3 : Mux  Inputs=2
  Mux9 : Mux  Inputs=2
  Position : Integrator  InitialConditionSource=external  ContinuousStateAttributes='position'
  Subsystem : Subsystem
  To Workspace : ToWorkspace  VariableName=simoutL  SampleTime=-1  SaveFormat=Structure With Time
  To Workspace1 : ToWorkspace  VariableName=simoutL1  SampleTime=-1  SaveFormat=Structure With Time
  To Workspace2 : ToWorkspace  VariableName=simoutL2  SampleTime=-1  SaveFormat=Structure With Time
  Velocity : Integrator  InitialConditionSource=external  ContinuousStateAttributes='velocity'
  Out5 : Outport
  Out2 : Outport  Port=2
  Out6 : Outport  Port=3
  Out3 : Outport  Port=4
  Out7 : Outport  Port=5
  Out4 : Outport  Port=6
  wires:
  In1/1 -> Mux8/3, Mux3/1  "ddxL"
  Demux1/2 -> Mux2/2  "dyL"
  Demux1/1 -> Mux2/1  "dxL"
  Demux1/3 -> Mux2/3  "dzL"
  Mux3/1 -> Velocity/1  "ddstates"
  Initial dstates/1(Init vel) -> Velocity/2
  Position/1 -> Demux2/1  "states"
  Demux2/2 -> Mux4/2  "yL"
  Demux2/1 -> Mux4/1  "xL"
  Demux2/3 -> Mux4/3  "zL"
  Initial states/1(Init vel) -> Position/2
  Demux2/4 -> Mux6/1  "phiL"
  Demux2/5 -> Mux6/2  "thetaL"
  Demux2/6 -> Mux6/3  "psiL"
  Velocity/1 -> Subsystem/2(In1), Demux1/1  "dstates"
  Mux2/1 -> Mux8/2, Out2/1  "dxL"
  Mux4/1 -> Mux8/1, Out5/1  "xL"
  In3/1 -> Mux3/2, Mux10/3  "dOmegaQ"
  Mux5/1 -> Mux10/2, Out4/1  "OmegaQ"
  Mux8/1 -> To Workspace/1
  Mux9/1 -> To Workspace1/1
  Mux10/1 -> To Workspace2/1
  In2/1 -> Subsystem/1(In2), Mux9/2, Out3/1  "OmegaL"
  Subsystem/1(Out1) -> Position/1
  Demux1/5 -> Mux5/2  "qL"
  Demux1/6 -> Mux5/3  "rL"
  Demux1/4 -> Mux5/1  "pL"
  In4/1 -> Direction Cosine Matrix to Rotation Angles/1  "R"
  Direction Cosine Matrix to Rotation Angles/1 -> Gain/1  "angleQ"
  Gain/1 -> Mux10/1, Out7/1  "angleQ"
  MATLAB Function/1(anglesL) -> Out6/1, Mux9/1  "anglesL"
  In5/1 -> MATLAB Function/1(q)  "q"

== system QRLsim/QR-Load Nonlinear model/R block ==
  note: R block
  Omega : Inport
  Integrator : Integrator  InitialCondition=R0  ContinuousStateAttributes='R'
  Saturation : Saturate  UpperLimit=1  LowerLimit=-1
  To Workspace4 : ToWorkspace  VariableName=simoutR  SampleTime=-1  SaveFormat=Structure With Time
  dR block : MATLAB Function  TreatAsAtomicUnit=on
  R : Outport
  wires:
  Integrator/1 -> Saturation/1  "R"
  dR block/1(dR) -> Integrator/1
  Omega/1 -> dR block/2(Omega)
  Saturation/1 -> dR block/1(R), To Workspace4/1, R/1  "R"

== system QRLsim/QR-Load Nonlinear model/T ==
  In2 : Inport
  Abs : Abs
  Constant : Constant  Value=g*e3
  Gain : Gain  Gain=mL
  Scope T : Scope
      settings: YMin=0  YMax=15  SaveName=ScopeData43
  Sum : Sum  Inputs=|++
  To Workspace1 : ToWorkspace  VariableName=simoutT  SampleTime=-1  SaveFormat=Structure With Time
  wires:
  Constant/1 -> Sum/2
  Abs/1 -> Scope T/1, To Workspace1/1
  Sum/1 -> Gain/1
  Gain/1 -> Abs/1
  In2/1 -> Sum/1  "ddxL"

== system QRLsim/QR-Load Nonlinear model/dOmegaQ block ==
  In1 : Inport
  Add : Sum  Inputs=-+
  Bus Selector : BusSelector  OutputSignals=OmegaQ,M
  Gain2 : Gain  Gain=inv(I)  Multiplication=Matrix(K*u)
  Subsystem1 : Subsystem
      mask Display: disp('\Omega \times I\Omega','texmode','on')
  dOmegaQ : Outport
  wires:
  In1/1 -> Bus Selector/1  "varQ"
  Bus Selector/1 -> Subsystem1/1(Omega)  "<OmegaQ>"
  Subsystem1/1(Out1) -> Add/1
  Add/1 -> Gain2/1  "J*dOmega"
  Bus Selector/2 -> Add/2  "<M>"
  Gain2/1 -> dOmegaQ/1  "dOmegaQ"

== system QRLsim/QR-Load Nonlinear model/omegarot block ==
  In3 : Inport
  In2 : Inport  Port=2
  In1 : Inport  Port=3
  Bus Selector2 : BusSelector  OutputSignals=sysvar.b,sysvar.d,sysvar.l  OutputAsBus=on
  Mux : Mux  Inputs=2
  Saturation : Saturate  UpperLimit=inf  LowerLimit=0  ZeroCross=off
  Sqrt : Sqrt  SaturateOnIntegerOverflow=on
  To Workspace3 : ToWorkspace  VariableName=simoutomegarot  SampleTime=-1  SaveFormat=Structure With Time
  fcnomega : MATLAB Function  TreatAsAtomicUnit=on
  Out1 : Outport
  Out2 : Outport  Port=2
  wires:
  In3/1 -> Bus Selector2/1
  In1/1 -> fcnomega/3(f)  "f"
  In2/1 -> fcnomega/2(M)  "M"
  Bus Selector2/1 -> fcnomega/1(var)  "var"
  Sqrt/1 -> Mux/2
  Saturation/1 -> Sqrt/1
  fcnomega/1(omegai) -> Mux/1, Saturation/1, Out1/1  "omegai"
  Mux/1 -> To Workspace3/1
  fcnomega/2(fi) -> Out2/1  "fi"

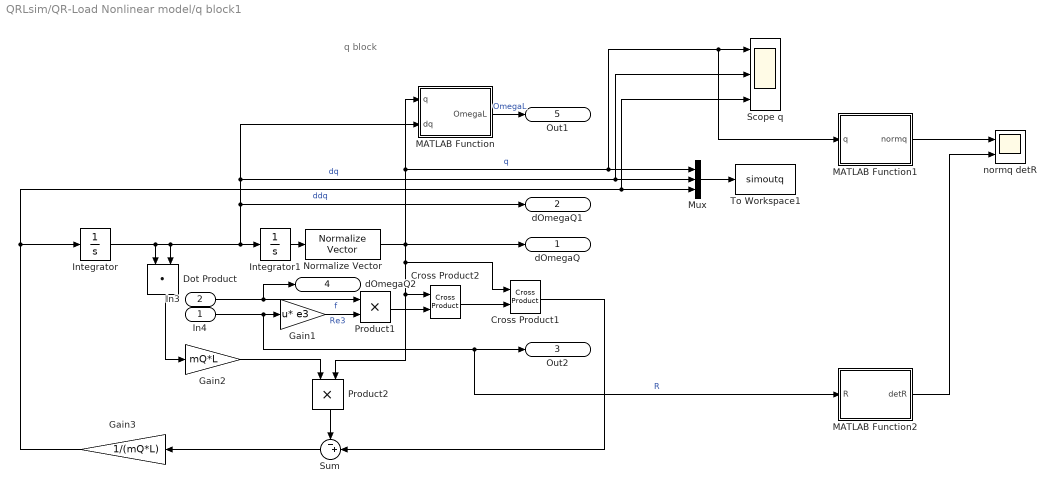
== system QRLsim/QR-Load Nonlinear model/q block1 ==
  note: q block
  In4 : Inport
  In3 : Inport  Port=2
  Cross Product1 : vrlib/Utilities/Cross Product
  Cross Product2 : vrlib/Utilities/Cross Product
  Dot Product : DotProduct  InputSameDT=on  OutDataTypeStr=Inherit: Inherit via internal rule
  Gain1 : Gain  Gain=e3  Multiplication=Matrix(u*K)
  Gain2 : Gain  Gain=mQ*L
  Gain3 : Gain  Gain=1/(mQ*L)
  Integrator : Integrator  InitialCondition=dq0  ContinuousStateAttributes='R'
  Integrator1 : Integrator  InitialCondition=q0  ContinuousStateAttributes='q'
  MATLAB Function : MATLAB Function  TreatAsAtomicUnit=on
  MATLAB Function1 : MATLAB Function  TreatAsAtomicUnit=on
  MATLAB Function2 : MATLAB Function  TreatAsAtomicUnit=on
  Mux : Mux  Inputs=3
  Normalize Vector : vrlib/Utilities/Normalize Vector  maxzero=0
  Product1 : Product
  Product2 : Product
  Scope q : Scope  NumInputPorts=3
      settings: ShowLegends=on  TimeRange=20  YMin=-1~-0.005~-0.75  YMax=0.1~0.04~1.75  SaveName=ScopeData39
  Sum : Sum  Inputs=-+|
  To Workspace1 : ToWorkspace  VariableName=simoutq  SampleTime=-1  SaveFormat=Structure With Time
  normq detR : Scope  NumInputPorts=2
      settings: YMin=-5~-5  YMax=5~5  SaveName=ScopeData29
  dOmegaQ : Outport
  dOmegaQ1 : Outport  Port=2
  Out2 : Outport  Port=3
  dOmegaQ2 : Outport  Port=4
  Out1 : Outport  Port=5
  wires:
  Dot Product/1 -> Gain2/1
  Gain3/1 -> Scope q/3, Mux/3, Integrator/1  "ddq"
  Integrator/1 -> Dot Product/1, Dot Product/2, Integrator1/1, dOmegaQ1/1, Scope q/2, Mux/2, MATLAB Function/2(dq)  "dq"
  In3/1 -> dOmegaQ2/1, Product1/1  "f"
  Gain1/1 -> Product1/2  "Re3"
  Product1/1 -> Cross Product2/2
  Cross Product2/1 -> Cross Product1/2
  Cross Product1/1 -> Sum/2
  Sum/1 -> Gain3/1
  In4/1 -> MATLAB Function2/1(R), Out2/1, Gain1/1  "R"
  Gain2/1 -> Product2/1
  Product2/1 -> Sum/1
  MATLAB Function/1(OmegaL) -> Out1/1  "OmegaL"
  Mux/1 -> To Workspace1/1
  Normalize Vector/1 -> MATLAB Function1/1(q), Scope q/1, Mux/1, MATLAB Function/1(q), dOmegaQ/1, Cross Product2/1, Product2/2, Cross Product1/1  "q"
  MATLAB Function1/1(normq) -> normq detR/1
  MATLAB Function2/1(detR) -> normq detR/2
  Integrator1/1 -> Normalize Vector/1

== system QRLsim/QR-Load Nonlinear model/var ddxL ==
  Bus Creator1 : BusCreator
  Cable length : Constant  Value=L
  Gravity Constant : Constant  Value=g
  Mass Load : Constant  Value=mL
  Mass QR : Constant  Value=mQ
  Var : Outport
  wires:
  Mass QR/1 -> Bus Creator1/1  "mQ"
  Cable length/1 -> Bus Creator1/4  "L"
  Mass Load/1 -> Bus Creator1/3  "mL"
  Bus Creator1/1 -> Var/1  "varddxL"
  Gravity Constant/1 -> Bus Creator1/2  "g"

== system QRLsim/QR-Load Nonlinear model/varQ ==
  Arm length : Constant  Value=l
  Bus Creator : BusCreator  Inputs=2
  Bus Creator1 : BusCreator  Inputs=8
  Cable length : Constant  Value=L
  Drag Factor : Constant  Value=d
  Gravity Constant : Constant  Value=g
  Mass QR : Constant  Value=mQ
  QR Inertia : Constant  Value=diag([Ixx,Iyy,Izz])
  Rotor Inertia : Constant  Value=Ir
  Thrust Factor : Constant  Value=b
  ctauf : Constant  Value=ctauf
      mask Display: disp('c_{\tau f}','texmode','on')
  Var : Outport
  wires:
  Gravity Constant/1 -> Bus Creator/2  "g"
  Bus Creator/1 -> Var/1  "varQ"
  Mass QR/1 -> Bus Creator1/1  "m"
  Arm length/1 -> Bus Creator1/6  "l"
  Rotor Inertia/1 -> Bus Creator1/5  "Ir"
  QR Inertia/1 -> Bus Creator1/2  "I"
  Bus Creator1/1 -> Bus Creator/1  "sysvar"
  Thrust Factor/1 -> Bus Creator1/3  "b"
  Drag Factor/1 -> Bus Creator1/4  "d"
  ctauf/1 -> Bus Creator1/7  "ctauf"
  Cable length/1 -> Bus Creator1/8  "lL"

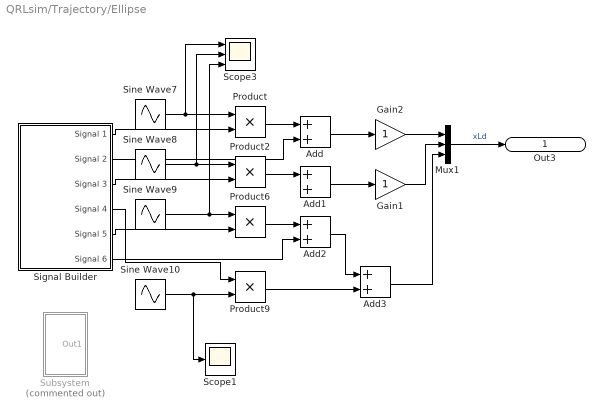
== system QRLsim/Trajectory/Ellipse ==
  Add{,1..3} (4 alike) : Sum
  Gain1 : Gain
  Gain2 : Gain
  Mux1 : Mux  Inputs=3
  Product{,2,6,9} (4 alike) : Product
  Scope1 : Scope
      settings: ShowLegends=on  YMin=-8  YMax=12  SaveName=ScopeData2
  Scope3 : Scope  NumInputPorts=3
      settings: TimeRange=25  YMin=0~0~0  YMax=2~0.5~0.5  SaveName=ScopeData23
  Signal Builder : Subsystem  Tag=STV Subsys  LoadFcn=sigbuilder_block('load');  StartFcn=sigbuilder_block('start');  StopFcn=sigbuilder_block('stop');  ClipboardFcn=sigbuilder_block('clipboard');  mask(Sigbuilder block){}
      mask help: Simulink:masks:SigbuilderBlock_MD
      mask init:
      | if ~strcmp(get_param(bdroot(gcbh),'SimulationStatus'),'stopped') tuvar = sigbuilder_block('maskInit'); end
      settings: CopyFcn=sigbuilder_block('copy');  DeleteFcn=sigbuilder_block('delete');  ModelCloseFcn=sigbuilder_block('modelClose');  PreSaveFcn=sigbuilder_block('preSave');  PauseFcn=sigbuilder_block('pause');  ContinueFcn=sigbuilder_block('continue');  NameChangeFcn=sigbuilder_block('namechange');  OpenFcn=sigbuilder_block('open',[-24 211.5 948 480 ]);  CloseFcn=sigbuilder_block('close');
      mask Display: plot(0, 0, 100, 100,[2, 2, 32, 32, 2], [68, 8, 8, 68, 68],[32, 2], [38, 38], [32, 19, 2],[53, 60, 44], [32, 17, 17, 2],[16, 16, 31, 31]);txt = getActiveGroup(gcbh);text(2, 100, txt,'verticalAlignment', 'top');
  Sine Wave10 : Sin  Amplitude=0.125  Bias=-.125  Frequency=2*pi/3  Phase=0.5*pi  SampleTime=0
  Sine Wave7 : Sin  Bias=1  Frequency=2*pi/20  Phase=pi  SampleTime=0
  Sine Wave8 : Sin  Amplitude=.4  Bias=.4  Frequency=2*pi/3  SampleTime=0
  Sine Wave9 : Sin  Amplitude=0.25  Frequency=2*pi/3  Phase=0.5*pi  SampleTime=0
  Subsystem : Subsystem  Commented=on
  Out3 : Outport
  wires:
  Add3/1 -> Mux1/3
  Gain1/1 -> Mux1/2
  Gain2/1 -> Mux1/1
  Sine Wave7/1 -> Product/1, Scope3/1
  Product/1 -> Add/1
  Signal Builder/1(Signal 1) -> Product/2
  Signal Builder/2(Signal 2) -> Add/2
  Signal Builder/3(Signal 3) -> Product2/2
  Signal Builder/5(Signal 5) -> Product6/2
  Product2/1 -> Add1/1
  Product6/1 -> Add2/1
  Add/1 -> Gain2/1
  Add1/1 -> Gain1/1
  Add2/1 -> Add3/1
  Sine Wave8/1 -> Product2/1, Scope3/2
  Sine Wave9/1 -> Scope3/3, Product6/1
  Mux1/1 -> Out3/1  "xLd"
  Signal Builder/6(Signal 6) -> Add2/2
  Signal Builder/4(Signal 4) -> Product9/1
  Sine Wave10/1 -> Scope1/1, Product9/2
  Product9/1 -> Add3/2

== system QRLsim/Trajectory/Path ==
  Manual Switch : ManualSwitch
  Sines : Subsystem
  Square : Subsystem
  Out3 : Outport
  wires:
  Square/1(Out1) -> Manual Switch/2
  Sines/1(Out1) -> Manual Switch/1
  Manual Switch/1 -> Out3/1  "xLd"

== system QRLsim/Trajectory/Step ==
  Manual Switch : ManualSwitch
  step1dir : Subsystem  mask{stept=stept, stepamp=stepamp}
      mask prompts: stept "Step time"; stepamp "Step Amplitude"
  step3dir : Subsystem
  Out2 : Outport
  wires:
  Manual Switch/1 -> Out2/1  "xLd"
  step3dir/1(Out1) -> Manual Switch/2
  step1dir/1(Out1) -> Manual Switch/1

== system QRLsim/Control Nonlinear Geometric/QRL Load Attitude Controller/Subsystem ==
  In1 : Inport
  In2 : Inport  Port=2
  In3 : Inport  Port=3
  Command Filter q1 : CF3/Command Filter  Integrator1_init=(mQ+mL)*(g*e3)  omega_n1=100  omega_n2=100  zeta=zeta_q
  Command Filter q2 : CF3/Command Filter  Integrator1_init=[0;-1;0]  omega_n1=100  omega_n2=100  zeta=zeta_q
  MATLAB Function : MATLAB Function  TreatAsAtomicUnit=on
  b3d1 : Outport
  b3d2 : Outport  Port=2
  wires:
  In1/1 -> Command Filter q1/1  "F"
  In2/1 -> Command Filter q2/1  "C"
  Command Filter q1/2 -> ?
  Command Filter q2/2 -> ?
  Command Filter q2/1 -> MATLAB Function/1(C)
  Command Filter q2/3 -> MATLAB Function/2(dC)
  Command Filter q2/4 -> MATLAB Function/3(ddC)
  Command Filter q1/1 -> MATLAB Function/5(F)
  Command Filter q1/3 -> MATLAB Function/6(dF)
  Command Filter q1/4 -> MATLAB Function/7(ddF)
  In3/1 -> MATLAB Function/4(b3c)  "b3c"
  MATLAB Function/1(dRc) -> b3d1/1  "dRc"
  MATLAB Function/2(ddRc) -> b3d2/1  "ddRc"

== system QRLsim/Control Nonlinear Geometric/QRL Load Attitude Controller/Subsystem2 ==
  Gain : Gain
  Mux2 : Mux  Inputs=3
  Product2 : Product
  Product5 : Product
  Product6 : Product
  Scope qd : Scope  NumInputPorts=2
      settings: YMin=-5~-5  YMax=5~5  SaveName=ScopeData38
  Sine Wave5 : Sin  Amplitude=.5  Frequency=2*pi/5  SampleTime=0
  Sine Wave6 : Sin  Amplitude=.5  Frequency=2*pi/5  Phase=pi/2  SampleTime=0
  Step2 : Step  Time=15  Before=1  After=0  SampleTime=0
  Step3 : Step  Time=15  Before=1  After=0  SampleTime=0
  Step4 : Step  Time=12.5  Before=-.85  After=-1  SampleTime=0
  qd : Outport
  wires:
  Sine Wave6/1 -> Product6/2
  Sine Wave5/1 -> Product5/2
  Step2/1 -> Product6/1, Product5/1
  Product5/1 -> Scope qd/2, Mux2/2
  Product6/1 -> Gain/1
  Gain/1 -> Product2/1
  Step3/1 -> Product2/2
  Product2/1 -> Scope qd/1, Mux2/1
  Mux2/1 -> qd/1  "qd"
  Step4/1 -> Mux2/3

== system QRLsim/Control Nonlinear Geometric/QRL QR Attitude Controller/Mterm Omegac ==
  Omega in : Inport
  R in : Inport  Port=2
  Rdes in : Inport  Port=3
  Rdes in1 : Inport  Port=4
  Rdes in2 : Inport  Port=5
  CFOmega : CommandFilter/Command Filter  Integrator1_init=0  omega_n=2*pi*15  zeta=.95
  Mux : Mux  Inputs=2
  Omegac block : MATLAB Function  TreatAsAtomicUnit=on
  Scope : Scope
      settings: ShowLegends=on  SaveName=ScopeData9
  Subsystem1 : Subsystem
      mask Display: disp('J_Q(\Omega^{hat}R^TR_c\Omega_c-R^TR_d\Omega\prime_c)','texmode','on')
  Terminator : Terminator
  Terminator1 : Terminator
  scope Omega Omegac : Scope  NumInputPorts=3
      settings: ShowLegends=on  YMin=-8~-5.5~-90  YMax=8~5.5~90  SaveName=ScopeData22
  Omegades : Outport
  M term : Outport  Port=2
  wires:
  Omega in/1 -> scope Omega Omegac/1, Subsystem1/2(In2)  "Omega"
  Omegac block/1(Omegac) -> CFOmega/1, scope Omega Omegac/2, Subsystem1/4(In4), Omegades/1  "Omegac"
  R in/1 -> Subsystem1/1(In1)  "R"
  Subsystem1/1(Out1) -> M term/1
  Rdes in/1 -> Subsystem1/3(In3), Omegac block/1(Rc)
  Rdes in2/1 -> Omegac block/3(ddRc)
  Rdes in1/1 -> Omegac block/2(dRc)
  CFOmega/2 -> Terminator/1
  CFOmega/1 -> Terminator1/1
  Mux/1 -> Scope/1
  Omegac block/2(dOmegac) -> scope Omega Omegac/3, Subsystem1/5(In5), Mux/2  "dOmegac"
  CFOmega/3 -> Mux/1  "CFdOmegac"

== system QRLsim/Control Nonlinear Geometric/QRL QR Attitude Controller/Subsystem2 ==
  Omega : Inport
  Cross Product : vrlib/Utilities/Cross Product
  I : Gain  Gain=I  Multiplication=Matrix(K*u)
  Out1 : Outport
  wires:
  Omega/1 -> Cross Product/1, I/1
  I/1 -> Cross Product/2
  Cross Product/1 -> Out1/1

== system QRLsim/QR-Load Nonlinear model/Integration Block/Initial dstates ==
  Bus Creator1 : BusCreator  Inputs=2
  OmegaQ0 : Constant  Value=[pQ0; qQ0; rQ0]
  dxL0 : Constant  Value=[dxL0;dyL0;dzL0]
  Init vel : Outport
  wires:
  dxL0/1 -> Bus Creator1/1  "dxL0"
  Bus Creator1/1 -> Init vel/1  "Init dstates"
  OmegaQ0/1 -> Bus Creator1/2  "OmegaQ0"

== system QRLsim/QR-Load Nonlinear model/Integration Block/Initial states ==
  Bus Creator1 : BusCreator  Inputs=2
  angleL0 : Constant  Value=[phiL0; thetaL0; psiL0]
  xL0 : Constant  Value=[xL0;yL0;zL0]
  Init vel : Outport
  wires:
  xL0/1 -> Bus Creator1/1  "xL0"
  Bus Creator1/1 -> Init vel/1  "Init states"
  angleL0/1 -> Bus Creator1/2  "angleL0"

== system QRLsim/QR-Load Nonlinear model/Integration Block/Subsystem ==
  In2 : Inport
  In1 : Inport  Port=2
  Demux3 : Demux  Outputs=6
  Mux11 : Mux
  Out1 : Outport
  wires:
  Mux11/1 -> Out1/1
  In1/1 -> Demux3/1
  Demux3/2 -> Mux11/2
  Demux3/1 -> Mux11/1
  Demux3/3 -> Mux11/3
  In2/1 -> Mux11/4

== system QRLsim/QR-Load Nonlinear model/dOmegaQ block/Subsystem1 ==
  Omega : Inport
  Cross Product : vrlib/Utilities/Cross Product
  I : Gain  Gain=I  Multiplication=Matrix(K*u)
  Out1 : Outport
  wires:
  Omega/1 -> Cross Product/1, I/1
  I/1 -> Cross Product/2
  Cross Product/1 -> Out1/1

== system QRLsim/Trajectory/Ellipse/Signal Builder ==
  Demux : Demux  Tag=STV Demux  Outputs=6
  FromWs : FromWorkspace  Tag=STV FromWs  VariableName=tuvar  SampleTime=0
      SigBuilderData=|
      | common.afterFinalStr = 'Extrapolate'
      | common.sampleTime = 0
      | dataSet.timeRange = [0 21]
      | dataSet.name = 'Group 1'
      | sbobj.Groups.Name = 'Group 1'
      | sbobj.Groups.Signals(1).Name = 'Signal 1'
      | sbobj.Groups.Signals(1).XData = [0 5 5 15 15 21]
      | sbobj.Groups.Signals(1).YData = [0 0 1 1 0 0]
      | sbobj.Groups.Signals(2).Name = 'Signal 2'
      | sbobj.Groups.Signals(2).XData = [0 15 15 21]
      | sbobj.Groups.Signals(2).YData = [0 0 2 2]
      | sbobj.Groups.Signals(3).Name = 'Signal 3'
      | sbobj.Groups.Signals(3).XData = [0 5.25 5.25 14.25 14.25 21]
      | sbobj.Groups.Signals(3).YData = [0 0 1 1 0 0]
      | sbobj.Groups.Signals(4).Name = 'Signal 4'
      | sbobj.Groups.Signals(4).XData = [0 1.5 1.5 21]
      | sbobj.Groups.Signals(4).YData = [1 1 0 0]
      | sbobj.Groups.Signals(5).Name = 'Signal 5'
      | sbobj.Groups.Signals(5).XData = [0 4.5 4.5 15 15 21]
      | sbobj.Groups.Signals(5).YData = [0 0 1 1 0 0]
      | sbobj.Groups.Signals(6).Name = 'Signal 6'
      | sbobj.Groups.Signals(6).XData = [0 1.5 1.5 4.5 4.5 15 15 21]
      | sbobj.Groups.Signals(6).YData = [0 0 -0.25 -0.25 0 0 0.25 0.25]
      | sbobj.Groups.TimeRange = [0 21]
  Signal 1 : Outport  Tag=STV Outport
  Signal 2 : Outport  Tag=STV Outport  Port=2
  Signal 3 : Outport  Tag=STV Outport  Port=3
  Signal 4 : Outport  Tag=STV Outport  Port=4
  Signal 5 : Outport  Tag=STV Outport  Port=5
  Signal 6 : Outport  Tag=STV Outport  Port=6
  wires:
  FromWs/1 -> Demux/1
  Demux/1 -> Signal 1/1
  Demux/2 -> Signal 2/1
  Demux/3 -> Signal 3/1
  Demux/4 -> Signal 4/1
  Demux/5 -> Signal 5/1
  Demux/6 -> Signal 6/1

== system QRLsim/Trajectory/Ellipse/Subsystem ==
  Constant : Constant  Value=0
  Constant1 : Constant
  Manual Switch1 : ManualSwitch
  Manual Switch2 : ManualSwitch
  Manual Switch3 : ManualSwitch
  Mux : Mux  Inputs=3
  Ramp : simulink/Sources/Ramp  slope=1/5  start=2  X0=0
  Ramp1 : simulink/Sources/Ramp  slope=0  start=0  X0=0
  Ramp2 : simulink/Sources/Ramp  slope=0  start=0  X0=0
  Sine Wave : Sin  Frequency=2*pi/T0  Phase=-pi/2  SampleTime=0
  Sine Wave3 : Sin  Frequency=2*pi/T0  SampleTime=0
  Sum2 : Sum  Inputs=|++
  Sum4 : Sum  Inputs=|++
  Out1 : Outport
  wires:
  Constant/1 -> Manual Switch1/2, Manual Switch3/2
  Sine Wave3/1 -> Sum2/2
  Manual Switch3/1 -> Mux/2
  Manual Switch2/1 -> Mux/3
  Manual Switch1/1 -> Mux/1
  Constant1/1 -> Manual Switch2/2
  Ramp1/1 -> Sum2/1
  Ramp2/1 -> Sum4/1
  Sum4/1 -> Manual Switch3/1
  Sine Wave/1 -> Sum4/2
  Ramp/1 -> Manual Switch1/1
  Sum2/1 -> Manual Switch2/1
  Mux/1 -> Out1/1

== system QRLsim/Trajectory/Path/Sines ==
  Manual Switch1 : ManualSwitch  CurrentSetting=0
  Manual Switch2 : ManualSwitch
  Sine diagonal : Subsystem
  Sine growing : Subsystem
  Sine up down : Subsystem
  Out1 : Outport
  wires:
  Sine diagonal/1(Out1) -> Manual Switch1/1
  Sine up down/1(Out2) -> Manual Switch1/2
  Manual Switch1/1 -> Manual Switch2/2
  Manual Switch2/1 -> Out1/1
  Sine growing/1(Out2) -> Manual Switch2/1

== system QRLsim/Trajectory/Path/Square ==
  CFSQ : CF3/Command Filter  Integrator1_init=0  omega_n1=2*pi*1.2*0.5  omega_n2=2*pi*1*.5  zeta=zeta_xL
  Constant : Constant  Value=0
  Gain : Gain  Gain=10
  Manual Switch1 : ManualSwitch
  Manual Switch2 : ManualSwitch  CurrentSetting=0
  Manual Switch3 : ManualSwitch
  Mux : Mux  Inputs=3
  Scope1 : Scope  NumInputPorts=3
      settings: ShowLegends=on  TimeRange=15  YMin=0~0~-1  YMax=1~1~1  SaveName=ScopeData7
  Signal Builder3 : Subsystem  Tag=STV Subsys  LoadFcn=sigbuilder_block('load');  StartFcn=sigbuilder_block('start');  StopFcn=sigbuilder_block('stop');  ClipboardFcn=sigbuilder_block('clipboard');  mask(Sigbuilder block){}
      mask help: Simulink:masks:SigbuilderBlock_MD
      mask init:
      | if ~strcmp(get_param(bdroot(gcbh),'SimulationStatus'),'stopped') tuvar = sigbuilder_block('maskInit'); end
      settings: CopyFcn=sigbuilder_block('copy');  DeleteFcn=sigbuilder_block('delete');  ModelCloseFcn=sigbuilder_block('modelClose');  PreSaveFcn=sigbuilder_block('preSave');  PauseFcn=sigbuilder_block('pause');  ContinueFcn=sigbuilder_block('continue');  NameChangeFcn=sigbuilder_block('namechange');  OpenFcn=sigbuilder_block('open',[181.5 90.75 999 399.75 ]);  CloseFcn=sigbuilder_block('close');
      mask Display: plot(0, 0, 100, 100,[2, 2, 32, 32, 2], [68, 8, 8, 68, 68],[32, 2], [38, 38], [32, 19, 2],[53, 60, 44], [32, 17, 17, 2],[16, 16, 31, 31]);txt = getActiveGroup(gcbh);text(2, 100, txt,'verticalAlignment', 'top');
  Out1 : Outport
  wires:
  Constant/1 -> Manual Switch2/2, Manual Switch3/2, Manual Switch1/2
  Manual Switch1/1 -> Mux/1
  Manual Switch2/1 -> Mux/3
  Manual Switch3/1 -> Mux/2
  Mux/1 -> Gain/1
  CFSQ/2 -> Scope1/2, Out1/1
  Signal Builder3/1(Signal 1) -> Manual Switch1/1
  Signal Builder3/2(Signal 2) -> Manual Switch3/1
  Gain/1 -> Scope1/1, CFSQ/1

== system QRLsim/Trajectory/Step/step1dir ==
  Add : Sum
  Gain : Gain  Gain=0
  Gain1 : Gain  Gain=stepamp
  Gain2 : Gain  Gain=0
  Mux2 : Mux  Inputs=3
  Product : Product
  Sine Wave : Sin  Amplitude=0.5  Bias=0.5  Frequency=2*pi/(2*stept)  Phase=1.5*pi  SampleTime=0
  Step : Step  Time=stept  Before=1  After=0  SampleTime=0
  Step1 : Step  Time=stept  SampleTime=0
  Out1 : Outport
  wires:
  Add/1 -> Gain2/1, Gain/1, Gain1/1
  Gain/1 -> Mux2/3
  Gain1/1 -> Mux2/2
  Gain2/1 -> Mux2/1
  Mux2/1 -> Out1/1  "xLd"
  Sine Wave/1 -> Product/1
  Product/1 -> Add/1
  Step/1 -> Product/2
  Step1/1 -> Add/2

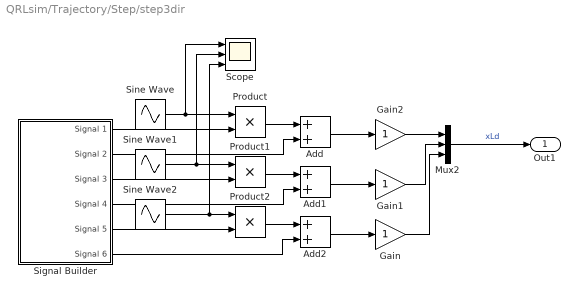
== system QRLsim/Trajectory/Step/step3dir ==
  Add : Sum
  Add1 : Sum
  Add2 : Sum
  Gain : Gain
  Gain1 : Gain
  Gain2 : Gain
  Mux2 : Mux  Inputs=3
  Product : Product
  Product1 : Product
  Product2 : Product
  Scope : Scope  NumInputPorts=3
      settings: YMin=-5~-5~-5  YMax=5~5~5  SaveName=ScopeData17
  Signal Builder : Subsystem  Tag=STV Subsys  LoadFcn=sigbuilder_block('load');  StartFcn=sigbuilder_block('start');  StopFcn=sigbuilder_block('stop');  ClipboardFcn=sigbuilder_block('clipboard');  mask(Sigbuilder block){}
      mask help: Simulink:masks:SigbuilderBlock_MD
      mask init:
      | if ~strcmp(get_param(bdroot(gcbh),'SimulationStatus'),'stopped') tuvar = sigbuilder_block('maskInit'); end
      settings: CopyFcn=sigbuilder_block('copy');  DeleteFcn=sigbuilder_block('delete');  ModelCloseFcn=sigbuilder_block('modelClose');  PreSaveFcn=sigbuilder_block('preSave');  PauseFcn=sigbuilder_block('pause');  ContinueFcn=sigbuilder_block('continue');  NameChangeFcn=sigbuilder_block('namechange');  OpenFcn=sigbuilder_block('open',[-18 126.75 550.5 507 ]);  CloseFcn=sigbuilder_block('close');
      mask Display: plot(0, 0, 100, 100,[2, 2, 32, 32, 2], [68, 8, 8, 68, 68],[32, 2], [38, 38], [32, 19, 2],[53, 60, 44], [32, 17, 17, 2],[16, 16, 31, 31]);txt = getActiveGroup(gcbh);text(2, 100, txt,'verticalAlignment', 'top');
  Sine Wave : Sin  Amplitude=0.5  Bias=0.5  Frequency=2*pi/6  Phase=7/6*pi  SampleTime=0
  Sine Wave1 : Sin  Amplitude=0.5  Bias=0.5  Frequency=2*pi/6  SampleTime=0
  Sine Wave2 : Sin  Amplitude=0.5  Bias=0.5  Frequency=2*pi/6  Phase=-7/6*pi  SampleTime=0
  Out1 : Outport
  wires:
  Gain/1 -> Mux2/3
  Gain1/1 -> Mux2/2
  Gain2/1 -> Mux2/1
  Mux2/1 -> Out1/1  "xLd"
  Sine Wave/1 -> Product/1, Scope/1
  Product/1 -> Add/1
  Signal Builder/1(Signal 1) -> Product/2
  Signal Builder/2(Signal 2) -> Add/2
  Signal Builder/3(Signal 3) -> Product1/2
  Signal Builder/5(Signal 5) -> Product2/2
  Product1/1 -> Add1/1
  Signal Builder/4(Signal 4) -> Add1/2
  Product2/1 -> Add2/1
  Signal Builder/6(Signal 6) -> Add2/2
  Add/1 -> Gain2/1
  Add1/1 -> Gain1/1
  Add2/1 -> Gain/1
  Sine Wave1/1 -> Product1/1, Scope/2
  Sine Wave2/1 -> Scope/3, Product2/1
